simulink model "Filters_Desing"  (R2022a)
settings: Solver=FixedStepAuto  StartTime=0.0  StopTime=10.0  FixedStep=1/100  RelTol=1e-3
libraries: simulink x8
settings Model: Creator=Mario  LastModifiedBy=Mario

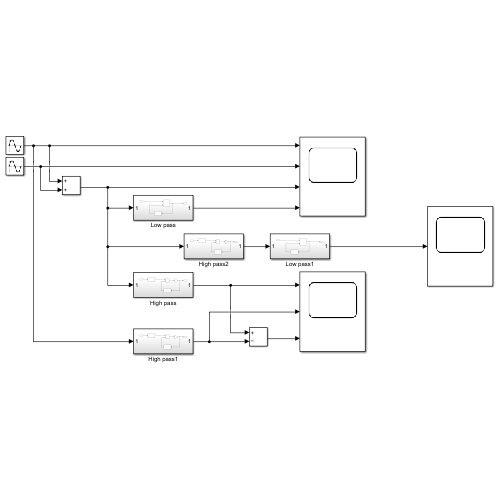
[thumbnail: Simulink's stored preview of the top-level diagram]
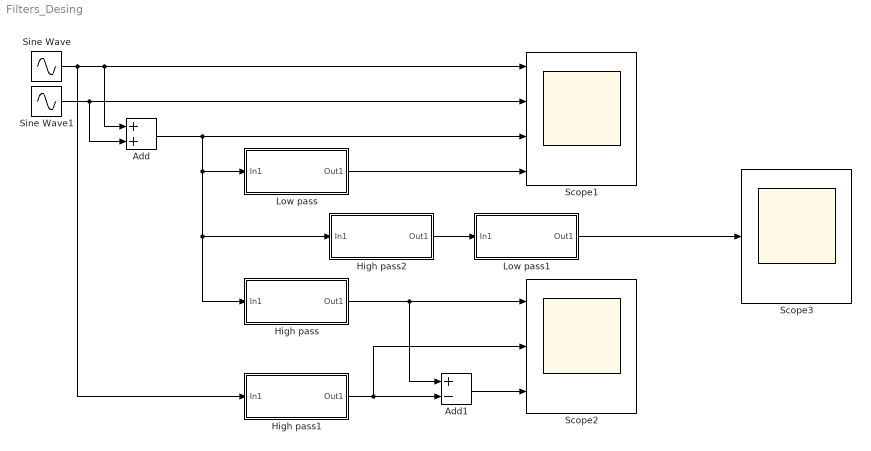
== system Filters_Desing ==
  Add : Sum
  Add1 : Sum  Inputs=+-
  High pass : Subsystem
  High pass1 : Subsystem
  High pass2 : Subsystem
  Low pass : Subsystem
  Low pass1 : Subsystem
  Scope1 : Scope  NumInputPorts=4
  Scope2 : Scope  NumInputPorts=3
  Scope3 : Scope
  Sine Wave : Sin  Amplitude=50  SampleTime=0
  Sine Wave1 : Sin  Amplitude=5  Frequency=100  SampleTime=0
  wires:
  Sine Wave/1 -> High pass1/1(In1), Add/1, Scope1/1
  Sine Wave1/1 -> Add/2, Scope1/2
  Low pass/1(Out1) -> Scope1/4
  Add/1 -> Low pass/1(In1), High pass2/1(In1), High pass/1(In1), Scope1/3
  High pass/1(Out1) -> Scope2/1, Add1/1
  Add1/1 -> Scope2/3
  High pass1/1(Out1) -> Add1/2, Scope2/2
  High pass2/1(Out1) -> Low pass1/1(In1)
  Low pass1/1(Out1) -> Scope3/1

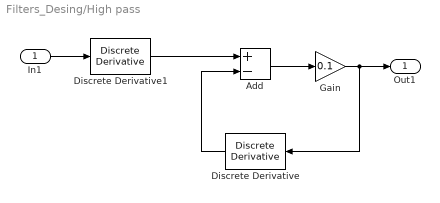
== system Filters_Desing/High pass ==
  In1 : Inport
  Add : Sum  Inputs=+-
  Discrete Derivative : simulink/Discrete/Discrete Derivative  gainval=1.0  ICPrevScaledInput=0.0  OutMin=[]  OutMax=[]  OutDataType=fixdt(1, 16)  OutScaling=2^-10  DoSatur=off
  Discrete Derivative1 : simulink/Discrete/Discrete Derivative  gainval=1.0  ICPrevScaledInput=0.0  OutMin=[]  OutMax=[]  OutDataType=fixdt(1, 16)  OutScaling=2^-10  DoSatur=off
  Gain : Gain  Gain=0.1
  Out1 : Outport
  wires:
  Add/1 -> Gain/1
  Gain/1 -> Discrete Derivative/1, Out1/1
  Discrete Derivative/1 -> Add/2
  Discrete Derivative1/1 -> Add/1
  In1/1 -> Discrete Derivative1/1

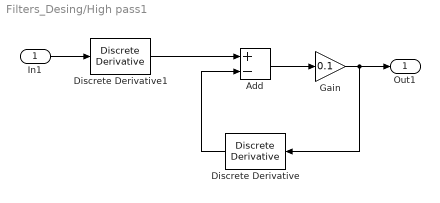
== system Filters_Desing/High pass1 ==
  In1 : Inport
  Add : Sum  Inputs=+-
  Discrete Derivative : simulink/Discrete/Discrete Derivative  gainval=1.0  ICPrevScaledInput=0.0  OutMin=[]  OutMax=[]  OutDataType=fixdt(1, 16)  OutScaling=2^-10  DoSatur=off
  Discrete Derivative1 : simulink/Discrete/Discrete Derivative  gainval=1.0  ICPrevScaledInput=0.0  OutMin=[]  OutMax=[]  OutDataType=fixdt(1, 16)  OutScaling=2^-10  DoSatur=off
  Gain : Gain  Gain=0.1
  Out1 : Outport
  wires:
  Add/1 -> Gain/1
  Gain/1 -> Discrete Derivative/1, Out1/1
  Discrete Derivative/1 -> Add/2
  Discrete Derivative1/1 -> Add/1
  In1/1 -> Discrete Derivative1/1

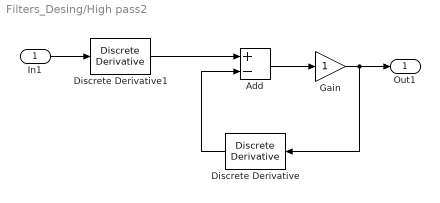
== system Filters_Desing/High pass2 ==
  In1 : Inport
  Add : Sum  Inputs=+-
  Discrete Derivative : simulink/Discrete/Discrete Derivative  gainval=1.0  ICPrevScaledInput=0.0  OutMin=[]  OutMax=[]  OutDataType=fixdt(1, 16)  OutScaling=2^-10  DoSatur=off
  Discrete Derivative1 : simulink/Discrete/Discrete Derivative  gainval=1.0  ICPrevScaledInput=0.0  OutMin=[]  OutMax=[]  OutDataType=fixdt(1, 16)  OutScaling=2^-10  DoSatur=off
  Gain : Gain
  Out1 : Outport
  wires:
  Add/1 -> Gain/1
  Gain/1 -> Discrete Derivative/1, Out1/1
  Discrete Derivative/1 -> Add/2
  Discrete Derivative1/1 -> Add/1
  In1/1 -> Discrete Derivative1/1

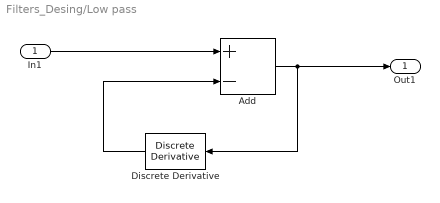
== system Filters_Desing/Low pass ==
  In1 : Inport
  Add : Sum  Inputs=+-
  Discrete Derivative : simulink/Discrete/Discrete Derivative  gainval=10  ICPrevScaledInput=0.0  OutMin=[]  OutMax=[]  OutDataType=fixdt(1, 16)  OutScaling=2^-10  DoSatur=off
  Out1 : Outport
  wires:
  In1/1 -> Add/1
  Discrete Derivative/1 -> Add/2
  Add/1 -> Discrete Derivative/1, Out1/1

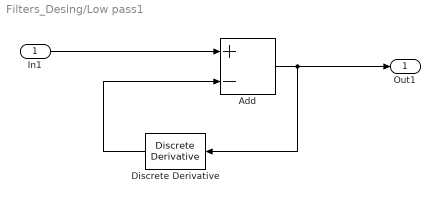
== system Filters_Desing/Low pass1 ==
  In1 : Inport
  Add : Sum  Inputs=+-
  Discrete Derivative : simulink/Discrete/Discrete Derivative  gainval=10  ICPrevScaledInput=0.0  OutMin=[]  OutMax=[]  OutDataType=fixdt(1, 16)  OutScaling=2^-10  DoSatur=off
  Out1 : Outport
  wires:
  In1/1 -> Add/1
  Discrete Derivative/1 -> Add/2
  Add/1 -> Discrete Derivative/1, Out1/1
